simulink model "Simulation_GSM_out"  (R2013b)
settings: Solver=ode45  StartTime=0.0  StopTime=20  MaxStep=1e-2  RelTol=1e-3
settings Model: Creator=am  LastModifiedBy=zp
settings OptimizationCC: ExpressionDepthLimit=2147483647
settings DebuggingCC: StateNameClashWarn=warning

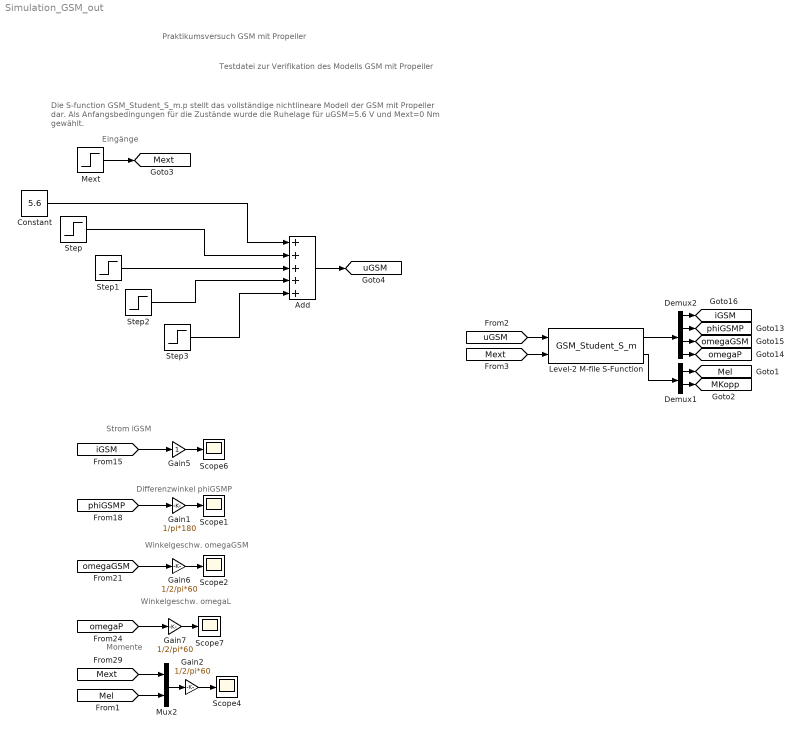
== system Simulation_GSM_out ==
  note: Strom iGSM
  note: Differenzwinkel phiGSMP
  note: Winkelgeschw. omegaGSM
  note: Winkelgeschw. omegaL
  note: Momente
  note: Testdatei zur Verifikation des Modells GSM mit Propeller
  note: Die S-function GSM_Student_S_m.p stellt das vollständige nichtlineare Modell
      | der GSM mit Propeller dar. Als Anfangsbedingungen für die Zustände wurde
      | die Ruhelage für uGSM=5.6 V und Mext=0 Nm gewählt.
  note: Praktikumsversuch GSM mit Propeller
  note: Eingänge
  Add : Sum  Inputs=+++++
  Constant : Constant  Value=5.6
  Demux1 : Demux  Outputs=2
  Demux2 : Demux
  Gain1 : Gain  Gain=1/pi*180
  Gain2 : Gain  Gain=1/2/pi*60
  Gain5 : Gain
  Gain6 : Gain  Gain=1/2/pi*60
  Gain7 : Gain  Gain=1/2/pi*60
  Level-2 M-file S-Function : M-S-Function  FunctionName=GSM_Student_S_m
  Mext : Step  Time=11  After=0.25  SampleTime=0
  Mux2 : Mux  Inputs=2
  Scope{1..2,4,6..7} (5 alike) : Scope
      Scope1 settings: YMin=-5.5  YMax=0.5
      Scope2 settings: YMin=-5.5  YMax=0.5
      Scope4 settings: YMin=0  YMax=1.4  SaveName=ScopeData3
      Scope6 settings: YMin=2  YMax=9  SaveName=ScopeData4
      Scope7 settings: YMin=-5.5  YMax=0.5  SaveName=ScopeData2
  Step : Step  Time=2  After=-1  SampleTime=0
  Step1 : Step  Time=5  After=2  SampleTime=0
  Step2 : Step  Time=8  After=-2  SampleTime=0
  Step3 : Step  Time=13  After=4  SampleTime=0
  tag scope: MKopp=global, Mel=global, Mext=global, iGSM=global, omegaGSM=global, omegaP=global, phiGSMP=global, uGSM=global
  wires:
  [uGSM] -> Level-2 M-file S-Function/1
  [Mext] -> Level-2 M-file S-Function/2
  Demux2/1 -> [iGSM]
  Demux2/2 -> [phiGSMP]
  Demux2/3 -> [omegaGSM]
  Demux2/4 -> [omegaP]
  Level-2 M-file S-Function/1 -> Demux2/1
  Level-2 M-file S-Function/2 -> Demux1/1
  Demux1/1 -> [Mel]
  Demux1/2 -> [MKopp]
  Mux2/1 -> Gain2/1
  Gain2/1 -> Scope4/1
  [iGSM] -> Gain5/1
  Gain5/1 -> Scope6/1
  Gain1/1 -> Scope1/1
  Gain6/1 -> Scope2/1
  Gain7/1 -> Scope7/1
  [Mext] -> Mux2/1
  [Mel] -> Mux2/2
  [phiGSMP] -> Gain1/1
  [omegaGSM] -> Gain6/1
  [omegaP] -> Gain7/1
  Mext/1 -> [Mext]
  Add/1 -> [uGSM]
  Step3/1 -> Add/5
  Step2/1 -> Add/4
  Step1/1 -> Add/3
  Step/1 -> Add/2
  Constant/1 -> Add/1
